simulink model "Trajactory_uav"  (R2022a)
settings: Solver=ode4  StartTime=0.0  StopTime=25  FixedStep=0.01  RelTol=1e-3
settings Model: Creator=liuwhale  LastModifiedBy=liuwhale
settings DebuggingCC: UnconnectedInputMsg=warning  UnconnectedOutputMsg=warning  UnconnectedLineMsg=warning
settings RTWCC: DLArmComputeVersion=19.05

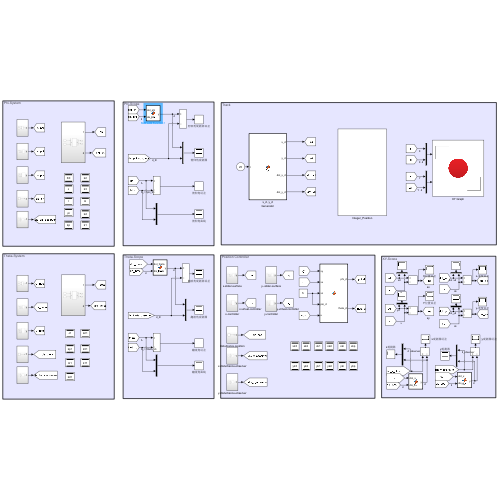
[thumbnail: Simulink's stored preview of the top-level diagram]
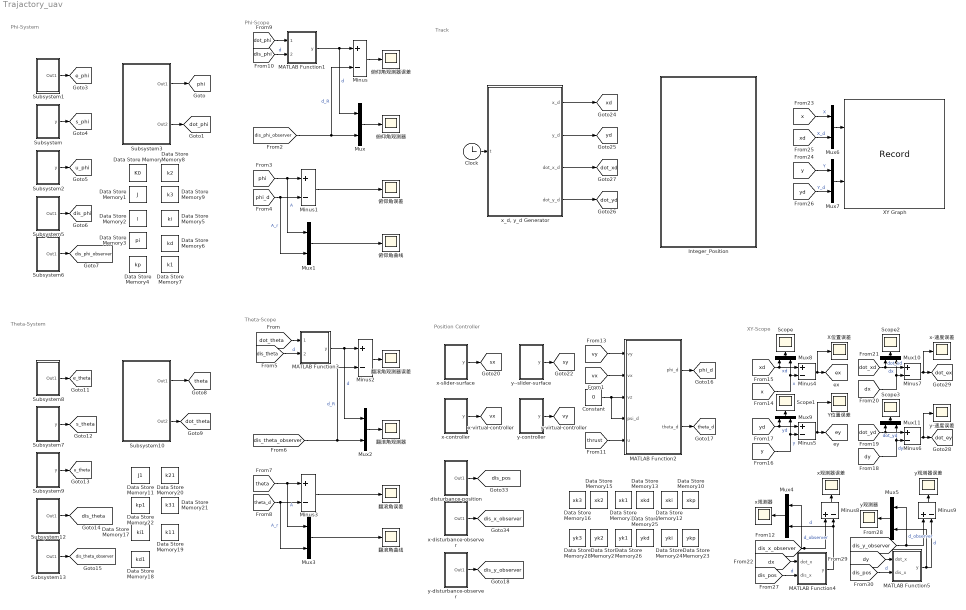
== system Trajactory_uav ==
  note: XY-Scope
  note: Track
  note: Position Controller
  note: Phi-Scope
  note: Phi-System
  note: Theta-System
  note: Theta-Scope
  Clock : Clock
  Constant : Constant  Value=0
  Data Store Memory : DataStoreMemory  DataStoreName=K0  ReadBeforeWriteMsg=warning  WriteAfterWriteMsg=warning  WriteAfterReadMsg=warning  InitialValue=0.01  ShowAdditionalParam=off  OutDataTypeStr=double
  Data Store Memory1 : DataStoreMemory  DataStoreName=J  ReadBeforeWriteMsg=warning  WriteAfterWriteMsg=warning  WriteAfterReadMsg=warning  InitialValue=0.005309688  ShowAdditionalParam=off  OutDataTypeStr=double
  Data Store Memory10 : DataStoreMemory  DataStoreName=xkp  ReadBeforeWriteMsg=warning  WriteAfterWriteMsg=warning  WriteAfterReadMsg=warning  InitialValue=1  ShowAdditionalParam=off  OutDataTypeStr=double
  Data Store Memory11 : DataStoreMemory  DataStoreName=J1  ReadBeforeWriteMsg=warning  WriteAfterWriteMsg=warning  WriteAfterReadMsg=warning  InitialValue=0.00577  ShowAdditionalParam=off  OutDataTypeStr=double
  Data Store Memory12 : DataStoreMemory  DataStoreName=xki  ReadBeforeWriteMsg=warning  WriteAfterWriteMsg=warning  WriteAfterReadMsg=warning  ShowAdditionalParam=off  OutDataTypeStr=double
  Data Store Memory13 : DataStoreMemory  DataStoreName=xkd  ReadBeforeWriteMsg=warning  WriteAfterWriteMsg=warning  WriteAfterReadMsg=warning  InitialValue=1  ShowAdditionalParam=off  OutDataTypeStr=double
  Data Store Memory14 : DataStoreMemory  DataStoreName=xk1  ReadBeforeWriteMsg=warning  WriteAfterWriteMsg=warning  WriteAfterReadMsg=warning  InitialValue=1  ShowAdditionalParam=off  OutDataTypeStr=double
  Data Store Memory15 : DataStoreMemory  DataStoreName=xk2  ReadBeforeWriteMsg=warning  WriteAfterWriteMsg=warning  WriteAfterReadMsg=warning  InitialValue=100  ShowAdditionalParam=off  OutDataTypeStr=double
  Data Store Memory16 : DataStoreMemory  DataStoreName=xk3  ReadBeforeWriteMsg=warning  WriteAfterWriteMsg=warning  WriteAfterReadMsg=warning  ShowAdditionalParam=off  OutDataTypeStr=double
  Data Store Memory17 : DataStoreMemory  DataStoreName=ki1  ReadBeforeWriteMsg=warning  WriteAfterWriteMsg=warning  WriteAfterReadMsg=warning  InitialValue=0.01  ShowAdditionalParam=off  OutDataTypeStr=double
  Data Store Memory18 : DataStoreMemory  DataStoreName=kd1  ReadBeforeWriteMsg=warning  WriteAfterWriteMsg=warning  WriteAfterReadMsg=warning  InitialValue=1  ShowAdditionalParam=off  OutDataTypeStr=double
  Data Store Memory19 : DataStoreMemory  DataStoreName=k11  ReadBeforeWriteMsg=warning  WriteAfterWriteMsg=warning  WriteAfterReadMsg=warning  InitialValue=1  ShowAdditionalParam=off  OutDataTypeStr=double
  Data Store Memory2 : DataStoreMemory  DataStoreName=l  ReadBeforeWriteMsg=warning  WriteAfterWriteMsg=warning  WriteAfterReadMsg=warning  InitialValue=0.33/sqrt(2)  ShowAdditionalParam=off  OutDataTypeStr=double
  Data Store Memory20 : DataStoreMemory  DataStoreName=k21  ReadBeforeWriteMsg=warning  WriteAfterWriteMsg=warning  WriteAfterReadMsg=warning  InitialValue=5  ShowAdditionalParam=off  OutDataTypeStr=double
  Data Store Memory21 : DataStoreMemory  DataStoreName=k31  ReadBeforeWriteMsg=warning  WriteAfterWriteMsg=warning  WriteAfterReadMsg=warning  InitialValue=0.001  ShowAdditionalParam=off  OutDataTypeStr=double
  Data Store Memory22 : DataStoreMemory  DataStoreName=kp1  ReadBeforeWriteMsg=warning  WriteAfterWriteMsg=warning  WriteAfterReadMsg=warning  InitialValue=30  ShowAdditionalParam=off  OutDataTypeStr=double
  Data Store Memory23 : DataStoreMemory  DataStoreName=ykp  ReadBeforeWriteMsg=warning  WriteAfterWriteMsg=warning  WriteAfterReadMsg=warning  InitialValue=1  ShowAdditionalParam=off  OutDataTypeStr=double
  Data Store Memory24 : DataStoreMemory  DataStoreName=yki  ReadBeforeWriteMsg=warning  WriteAfterWriteMsg=warning  WriteAfterReadMsg=warning  ShowAdditionalParam=off  OutDataTypeStr=double
  Data Store Memory25 : DataStoreMemory  DataStoreName=ykd  ReadBeforeWriteMsg=warning  WriteAfterWriteMsg=warning  WriteAfterReadMsg=warning  InitialValue=1  ShowAdditionalParam=off  OutDataTypeStr=double
  Data Store Memory26 : DataStoreMemory  DataStoreName=yk1  ReadBeforeWriteMsg=warning  WriteAfterWriteMsg=warning  WriteAfterReadMsg=warning  InitialValue=1  ShowAdditionalParam=off  OutDataTypeStr=double
  Data Store Memory27 : DataStoreMemory  DataStoreName=yk2  ReadBeforeWriteMsg=warning  WriteAfterWriteMsg=warning  WriteAfterReadMsg=warning  InitialValue=100  ShowAdditionalParam=off  OutDataTypeStr=double
  Data Store Memory28 : DataStoreMemory  DataStoreName=yk3  ReadBeforeWriteMsg=warning  WriteAfterWriteMsg=warning  WriteAfterReadMsg=warning  ShowAdditionalParam=off  OutDataTypeStr=double
  Data Store Memory3 : DataStoreMemory  DataStoreName=pi  ReadBeforeWriteMsg=warning  WriteAfterWriteMsg=warning  WriteAfterReadMsg=warning  InitialValue=3.1415926  ShowAdditionalParam=off  OutDataTypeStr=double
  Data Store Memory4 : DataStoreMemory  DataStoreName=kp  ReadBeforeWriteMsg=warning  WriteAfterWriteMsg=warning  WriteAfterReadMsg=warning  InitialValue=30  ShowAdditionalParam=off  OutDataTypeStr=double
  Data Store Memory5 : DataStoreMemory  DataStoreName=ki  ReadBeforeWriteMsg=warning  WriteAfterWriteMsg=warning  WriteAfterReadMsg=warning  InitialValue=0.01  ShowAdditionalParam=off  OutDataTypeStr=double
  Data Store Memory6 : DataStoreMemory  DataStoreName=kd  ReadBeforeWriteMsg=warning  WriteAfterWriteMsg=warning  WriteAfterReadMsg=warning  InitialValue=1  ShowAdditionalParam=off  OutDataTypeStr=double
  Data Store Memory7 : DataStoreMemory  DataStoreName=k1  ReadBeforeWriteMsg=warning  WriteAfterWriteMsg=warning  WriteAfterReadMsg=warning  InitialValue=1  ShowAdditionalParam=off  OutDataTypeStr=double
  Data Store Memory8 : DataStoreMemory  DataStoreName=k2  ReadBeforeWriteMsg=warning  WriteAfterWriteMsg=warning  WriteAfterReadMsg=warning  InitialValue=5  ShowAdditionalParam=off  OutDataTypeStr=double
  Data Store Memory9 : DataStoreMemory  DataStoreName=k3  ReadBeforeWriteMsg=warning  WriteAfterWriteMsg=warning  WriteAfterReadMsg=warning  InitialValue=0.001  ShowAdditionalParam=off  OutDataTypeStr=double
  Integer_Position : Subsystem
  MATLAB Function1 : MATLAB Function  TreatAsAtomicUnit=on
  MATLAB Function2 : MATLAB Function  TreatAsAtomicUnit=on
  MATLAB Function3 : MATLAB Function  TreatAsAtomicUnit=on
  MATLAB Function4 : MATLAB Function  TreatAsAtomicUnit=on
  MATLAB Function5 : MATLAB Function  TreatAsAtomicUnit=on
  Minus{,1..9} (10 alike) : Sum  Inputs=+-
  Mux{,1..11} (12 alike) : Mux  Inputs=2
  Scope{,1..3} (4 alike) : Scope
  Subsystem : Subsystem
  Subsystem1 : Subsystem
  Subsystem10 : Subsystem
  Subsystem12 : Subsystem
  Subsystem13 : Subsystem
  Subsystem2 : Subsystem
  Subsystem3 : Subsystem
  Subsystem5 : Subsystem
  Subsystem6 : Subsystem
  Subsystem7 : Subsystem
  Subsystem8 : Subsystem
  Subsystem9 : Subsystem
  XY Graph : Record  RecordToWorkspace=on  FileSettingsInternal="{\"entries\":[{\"content\":{\"excelSettings\":{\"content\":{},\"type\":\"Streamout.ExcelSettings\"}},\"type\":\"Streamout.FileSettingStorage\",\"uuid\":\"cb515a56-81c6-47bd-8ef5-eec051ca2d3d\"}],\"packageUris\":[\"http://schema.mathworks.com/mf0/streamout_blocks/R2020a\"],\"version\":\"1.0\"}"  Layout=[1 1]  SignalsInternal="{\"entries\":[{\"content\":{\"signals\":[{\"content\":{\"blockPath\":[\"Trajactory_uav/XY Graph\"],\"channel\":[],\"dimensions\":[2],\"domain\":\"Trajactory_uav/XY Graph\",\"hasChildren\":true,\"lineColor\":\"#0072bd\",\"plots\":[],\"port\":1,\"sid\":[\"\"],\"signalID\":412,\"signalName\":\"Mux6\"},\"type\":\"RecordBlkView.Signal\",\"uuid\":\"3dcd1e12-03f3-405f-916b-5c80faeb8bef\"},{\"content\":{\"blockPath\":[\"Trajactory_uav/XY Graph\"],\"channel\":[1],\"dimensions\":[2],\"domain\":\"Trajactory_uav/XY Graph\",\"lineColor\":\"#d95319\",\"parentID\":412,\"plots\":[1],\"port\":1,\"sid\":[\"\"],\"signalID\":413,\"signalName\":\"Mux6\"},\"type\":\"RecordBlkView.Signal\",\"uuid\":\"11d0947b-d576-4e4d-964d-e577cf2fd32e\"},{\"content\":{\"blockPath\":[\"Trajactory_uav/XY Graph\"],\"channel\":[],\"dimensions\":[2],\"domain\":\"Trajactory_uav/XY Graph\",\"hasChildren\":true,\"lineColor\":\"#edb120\",\"plots\":[],\"port\":2,\"sid\":[\"\"],\"signalID\":417,\"signalName\":\"Mux7\"},\"type\":\"RecordBlkView.Signal\",\"uuid\":\"3379d438-6583-47b9-80cc-092c1c32a13f\"},{\"content\":{\"blockPath\":[\"Trajactory_uav/XY Graph\"],\"channel\":[1],\"dimensions\":[2],\"domain\":\"Trajactory_uav/XY Graph\",\"lineColor\":\"#0072bd\",\"parentID\":417,\"plots\":[1],\"port\":2,\"sid\":[\"\"],\"signalID\":418,\"signalName\":\"Mux7\"},\"type\":\"RecordBlkView.Signal\",\"uuid\":\"342c55b0-3c25-4b78-9321-4ec9a5f92615\"},{\"content\":{\"blockPath\":[\"Trajactory_uav/XY Graph\"],\"channel\":[2],\"dimensions\":[2],\"domain\":\"Trajactory_uav/XY Graph\",\"lineColor\":\"#ff6929\",\"parentID\":412,\"plots\":[1],\"port\":1,\"sid\":[\"\"],\"signalID\":431,\"signalName\":\"Mux6\"},\"type\":\"RecordBlkView.Signal\",\"uuid\":\"21f03ca2-9128-487a-99db-9b74c0302f26\"},{\"content\":{\"blockPath\":[\"Trajactory_uav/XY Graph\"],\"channel\":[2],\"dimensions\":[2],\"domain\":\"Trajactory_uav/XY Graph\",\"lineColor\":\"#d95319\",\"parentID\":417,\"plots\":[1],\"port\":2,\"sid\":[\"\"],\"signalID\":432,\"signalName\":\"Mux7\"},\"type\":\"RecordBlkView.Signal\",\"uuid\":\"e9a965a2-3574-4d7b-b30c-2ed9b65f5195\"}]},\"type\":\"RecordBlkView.InputSignals\",\"uuid\":\"7f01d153-5e7e-44f9-865f-c21572bec30b\"}],\"packageUris\":[\"http://schema.mathworks.com/mf0/streamout_blocks/R2020a\"],\"version\":\"1.0\"}"  VisualizationBindings="{\"xyplotplugin\":{\"info\":[{\"series\":[{\"bindingParametersList\":[{\"parameter\":\"X-Axis\",\"signalID\":413,\"signalName\":\"Mux6(1)\"},{\"parameter\":\"Y-Axis\",\"signalID\":418,\"signalName\":\"Mux7(1)\"}],\"seriesID\":8627},{\"bindingParametersList\":[{\"parameter\":\"X-Axis\",\"signalID\":431,\"signalName\":\"Mux6(2)\"},{\"parameter\":\"Y-Axis\",\"signalID\":432,\"signalName\":\"Mux7(2)\"}],\"seriesID\":43199}],\"subplotID\":1}]}}"  CompatibilityTag=XY
  X位置误差 : Scope
  Y位置误差 : Scope
  disturbance-position : Subsystem
  x-controller : Subsystem
  x-disturbance-observer : Subsystem
  x-slider-surface : Subsystem
  x-速度误差 : Scope
  "x_d, y_d Generator" : MATLAB Function  TreatAsAtomicUnit=on
  x观测器 : Scope
  x观测器误差 : Scope
  y--slider-surface : Subsystem
  y-controller : Subsystem
  y-disturbance-observer : Subsystem
  y-速度误差 : Scope
  y观测器 : Scope
  y观测器误差 : Scope
  俯仰角曲线 : Scope
  俯仰角观测器 : Scope
  俯仰角观测器误差 : Scope
  俯仰角误差 : Scope
  翻滚角曲线 : Scope
  翻滚角观测器 : Scope
  翻滚角观测器误差 : Scope
  翻滚角误差 : Scope
  tag scope: dis_phi=global, dis_phi_observer=global, dis_pos=global, dis_theta=global, dis_theta_observer=global, dis_x_observer=global, dis_y_observer=global, dot_ex=global, dot_ey=global, dot_phi=global, dot_theta=global, dot_xd=global, dot_yd=global, e_phi=global, e_theta=global, ex=global, ey=global, phi=global, phi_d=global, s_phi=global, s_theta=global, sx=global, sy=global, theta=global, theta_d=global, u_phi=global, u_theta=global, vx=global, vy=global, xd=global, yd=global
  wires:
  Subsystem/1(y) -> [s_phi]
  Subsystem1/1(Out1) -> [e_phi]
  Subsystem2/1(y) -> [u_phi]
  Subsystem3/2(Out2) -> [dot_phi]
  Subsystem5/1(Out1) -> [dis_phi]
  Subsystem6/1(Out1) -> [dis_phi_observer]
  MATLAB Function1/1(y) -> Mux/1, Minus/1  "d"
  [dis_phi_observer] -> Minus/2, Mux/2  "d_R"
  Minus/1 -> 俯仰角观测器误差/1
  Mux/1 -> 俯仰角观测器/1
  Minus1/1 -> 俯仰角误差/1
  Mux1/1 -> 俯仰角曲线/1
  [phi_d] -> Mux1/2, Minus1/2  "A_r"
  [phi] -> Mux1/1, Minus1/1  "A"
  Subsystem8/1(Out1) -> [e_theta]
  Subsystem12/1(Out1) -> [dis_theta]
  Subsystem13/1(Out1) -> [dis_theta_observer]
  Subsystem7/1(y) -> [s_theta]
  Subsystem10/2(Out2) -> [dot_theta]
  Subsystem9/1(y) -> [u_theta]
  Minus2/1 -> 翻滚角观测器误差/1
  [theta] -> Mux3/1, Minus3/1  "A"
  [dis_theta_observer] -> Minus2/2, Mux2/2  "d_R"
  MATLAB Function3/1(y) -> Mux2/1, Minus2/1  "d"
  [theta_d] -> Mux3/2, Minus3/2  "A_r"
  Minus3/1 -> 翻滚角误差/1
  Mux3/1 -> 翻滚角曲线/1
  Mux2/1 -> 翻滚角观测器/1
  [dot_theta] -> MATLAB Function3/1(dot_theta)
  [dis_phi] -> MATLAB Function1/2(dis_phi)  "d"
  [dot_phi] -> MATLAB Function1/1(dot_phi)
  "x_d, y_d Generator"/2(y_d) -> [yd]
  "x_d, y_d Generator"/4(dot_y_d) -> [dot_yd]
  "x_d, y_d Generator"/3(dot_x_d) -> [dot_xd]
  Subsystem3/1(Out1) -> [phi]
  Subsystem10/1(Out1) -> [theta]
  Minus5/1 -> Y位置误差/1, [ey]
  [yd] -> Mux9/1, Minus5/1  "yd"
  [dx] -> Mux10/2, Minus7/2  "dx"
  [dy] -> Mux11/2, Minus6/2  "dy"
  Minus7/1 -> x-速度误差/1, [dot_ex]
  [x] -> Mux8/2, Minus4/2  "x"
  [dot_xd] -> Minus7/1, Mux10/1  "dot_xd"
  Minus6/1 -> y-速度误差/1, [dot_ey]
  [xd] -> Minus4/1, Mux8/1  "xd"
  Minus4/1 -> X位置误差/1, [ex]
  [dot_yd] -> Mux11/1, Minus6/1  "dot_yd"
  MATLAB Function2/2(theta_d) -> [theta_d]
  MATLAB Function2/1(phi_d) -> [phi_d]
  [thrust] -> MATLAB Function2/5(u)
  Constant/1 -> MATLAB Function2/3(vz), MATLAB Function2/4(psi_d)
  y-controller/1(y) -> [vy]
  x-controller/1(y) -> [vx]
  y--slider-surface/1(y) -> [sy]
  x-slider-surface/1(y) -> [sx]
  Clock/1 -> "x_d, y_d Generator"/1(t)
  "x_d, y_d Generator"/1(x_d) -> [xd]
  [vy] -> MATLAB Function2/1(vy)
  [vx] -> MATLAB Function2/2(vx)
  [dis_theta] -> MATLAB Function3/2(dis_theta)  "d"
  x-disturbance-observer/1(Out1) -> [dis_x_observer]
  disturbance-position/1(Out1) -> [dis_pos]
  [dx] -> MATLAB Function4/1(dot_x)
  [dis_x_observer] -> Minus8/1, Mux4/1  "d_observer"
  Mux4/1 -> x观测器/1
  MATLAB Function4/1(y) -> Mux4/2, Minus8/2  "d"
  Minus8/1 -> x观测器误差/1
  [dis_pos] -> MATLAB Function4/2(dis_x)  "d"
  y-disturbance-observer/1(Out1) -> [dis_y_observer]
  [dis_pos] -> MATLAB Function5/2(dis_x)  "d"
  [dy] -> MATLAB Function5/1(dot_x)
  MATLAB Function5/1(y) -> Minus9/2, Mux5/2  "d"
  Mux5/1 -> y观测器/1
  [dis_y_observer] -> Minus9/1, Mux5/1  "d_observer"
  Minus9/1 -> y观测器误差/1
  [yd] -> Mux7/2  "Y_d"
  Mux7/1 -> XY Graph/2
  [y] -> Mux7/1  "Y"
  Mux6/1 -> XY Graph/1
  [xd] -> Mux6/2  "X_d"
  [x] -> Mux6/1  "X"
  Mux8/1 -> Scope/1
  Mux9/1 -> Scope1/1
  [y] -> Mux9/2, Minus5/2  "y"
  Mux10/1 -> Scope2/1
  Mux11/1 -> Scope3/1

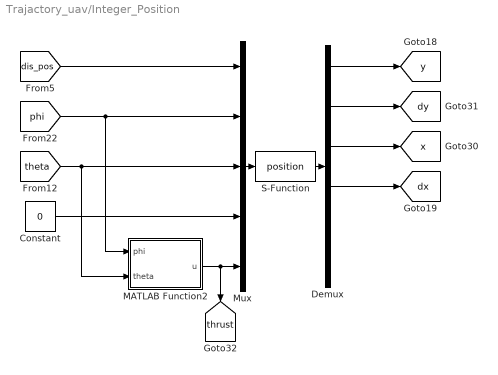
== system Trajactory_uav/Integer_Position ==
  Constant : Constant  Value=0
  Demux : Demux  Outputs=6
  MATLAB Function2 : MATLAB Function  TreatAsAtomicUnit=on
  Mux : Mux  Inputs=5
  S-Function : S-Function  FunctionName=position  SFunctionDeploymentMode=off  EnableBusSupport=off
  tag scope: dx=global, dy=global, thrust=global, x=global, y=global
  wires:
  [theta] -> Mux/3, MATLAB Function2/2(theta)
  [phi] -> Mux/2, MATLAB Function2/1(phi)
  MATLAB Function2/1(u) -> [thrust], Mux/5
  Mux/1 -> S-Function/1
  S-Function/1 -> Demux/1
  Constant/1 -> Mux/4
  Demux/3 -> [x]
  Demux/1 -> [y]
  Demux/2 -> [dy]
  Demux/4 -> [dx]
  [dis_pos] -> Mux/1

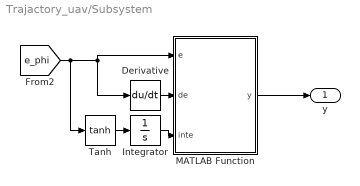
== system Trajactory_uav/Subsystem ==
  Derivative : Derivative
  Integrator : Integrator
  MATLAB Function : MATLAB Function  TreatAsAtomicUnit=on
  Tanh : Trigonometry  Operator=tanh
  y : Outport
  wires:
  [e_phi] -> Tanh/1, Derivative/1, MATLAB Function/1(e)
  Derivative/1 -> MATLAB Function/2(de)
  Integrator/1 -> MATLAB Function/3(inte)
  MATLAB Function/1(y) -> y/1
  Tanh/1 -> Integrator/1

== system Trajactory_uav/Subsystem1 ==
  Minus : Sum  Inputs=-+
  Out1 : Outport
  wires:
  [phi] -> Minus/1
  [phi_d] -> Minus/2
  Minus/1 -> Out1/1

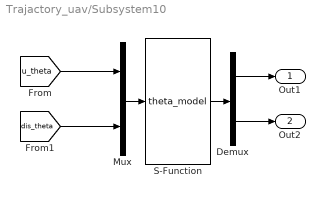
== system Trajactory_uav/Subsystem10 ==
  Demux : Demux  Outputs=2
  Mux : Mux  Inputs=2
  S-Function : S-Function  FunctionName=theta_model  SFunctionDeploymentMode=off  EnableBusSupport=off
  Out1 : Outport
  Out2 : Outport  Port=2
  wires:
  Mux/1 -> S-Function/1
  [u_theta] -> Mux/1
  S-Function/1 -> Demux/1
  Demux/1 -> Out1/1
  Demux/2 -> Out2/1
  [dis_theta] -> Mux/2

== system Trajactory_uav/Subsystem12 ==
  Sine Wave : Sin  Frequency=100  SampleTime=0
  Out1 : Outport
  wires:
  Sine Wave/1 -> Out1/1

== system Trajactory_uav/Subsystem13 ==
  Mux : Mux  Inputs=2
  S-Function : S-Function  FunctionName=DO_theta  SFunctionDeploymentMode=off  EnableBusSupport=off
  Out1 : Outport
  wires:
  S-Function/1 -> Out1/1
  [u_theta] -> Mux/1
  [dot_theta] -> Mux/2
  Mux/1 -> S-Function/1

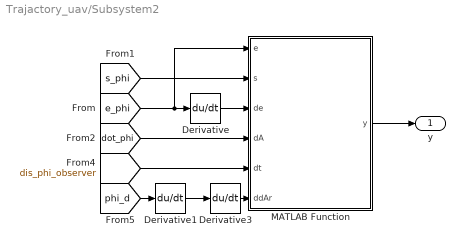
== system Trajactory_uav/Subsystem2 ==
  Derivative : Derivative
  Derivative1 : Derivative
  Derivative3 : Derivative
  MATLAB Function : MATLAB Function  TreatAsAtomicUnit=on
  y : Outport
  wires:
  [phi_d] -> Derivative1/1
  [s_phi] -> MATLAB Function/2(s)
  Derivative3/1 -> MATLAB Function/6(ddAr)
  [e_phi] -> MATLAB Function/1(e), Derivative/1
  MATLAB Function/1(y) -> y/1
  [dot_phi] -> MATLAB Function/4(dA)
  Derivative/1 -> MATLAB Function/3(de)
  Derivative1/1 -> Derivative3/1
  [dis_phi_observer] -> MATLAB Function/5(dt)

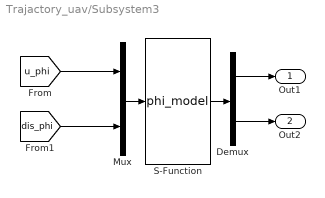
== system Trajactory_uav/Subsystem3 ==
  Demux : Demux  Outputs=2
  Mux : Mux  Inputs=2
  S-Function : S-Function  FunctionName=phi_model  SFunctionDeploymentMode=off  EnableBusSupport=off
  Out1 : Outport
  Out2 : Outport  Port=2
  wires:
  Mux/1 -> S-Function/1
  [u_phi] -> Mux/1
  S-Function/1 -> Demux/1
  Demux/1 -> Out1/1
  Demux/2 -> Out2/1
  [dis_phi] -> Mux/2

== system Trajactory_uav/Subsystem5 ==
  Sine Wave : Sin  Frequency=100  SampleTime=0
  Out1 : Outport
  wires:
  Sine Wave/1 -> Out1/1

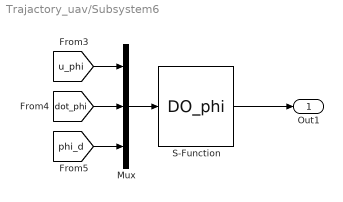
== system Trajactory_uav/Subsystem6 ==
  Mux : Mux  Inputs=3
  S-Function : S-Function  FunctionName=DO_phi  SFunctionDeploymentMode=off  EnableBusSupport=off
  Out1 : Outport
  wires:
  S-Function/1 -> Out1/1
  [u_phi] -> Mux/1
  [phi_d] -> Mux/3
  [dot_phi] -> Mux/2
  Mux/1 -> S-Function/1

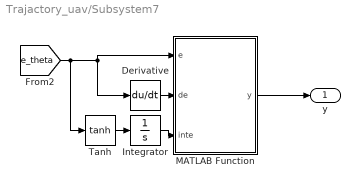
== system Trajactory_uav/Subsystem7 ==
  Derivative : Derivative
  Integrator : Integrator
  MATLAB Function : MATLAB Function  TreatAsAtomicUnit=on
  Tanh : Trigonometry  Operator=tanh
  y : Outport
  wires:
  [e_theta] -> Tanh/1, Derivative/1, MATLAB Function/1(e)
  Derivative/1 -> MATLAB Function/2(de)
  Integrator/1 -> MATLAB Function/3(inte)
  MATLAB Function/1(y) -> y/1
  Tanh/1 -> Integrator/1

== system Trajactory_uav/Subsystem8 ==
  Minus : Sum  Inputs=-+
  Out1 : Outport
  wires:
  [theta] -> Minus/1
  [theta_d] -> Minus/2
  Minus/1 -> Out1/1

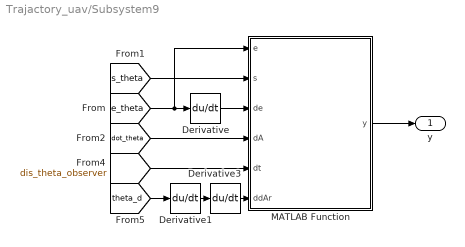
== system Trajactory_uav/Subsystem9 ==
  Derivative : Derivative
  Derivative1 : Derivative
  Derivative3 : Derivative
  MATLAB Function : MATLAB Function  TreatAsAtomicUnit=on
  y : Outport
  wires:
  [theta_d] -> Derivative1/1
  [s_theta] -> MATLAB Function/2(s)
  Derivative3/1 -> MATLAB Function/6(ddAr)
  [e_theta] -> MATLAB Function/1(e), Derivative/1
  MATLAB Function/1(y) -> y/1
  Derivative/1 -> MATLAB Function/3(de)
  Derivative1/1 -> Derivative3/1
  [dis_theta_observer] -> MATLAB Function/5(dt)
  [dot_theta] -> MATLAB Function/4(dA)

== system Trajactory_uav/disturbance-position ==
  Sine Wave : Sin  SampleTime=0
  Out1 : Outport
  wires:
  Sine Wave/1 -> Out1/1

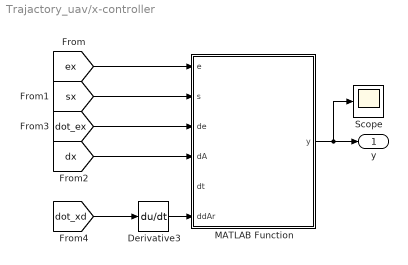
== system Trajactory_uav/x-controller ==
  Derivative3 : Derivative
  MATLAB Function : MATLAB Function  TreatAsAtomicUnit=on
  Scope : Scope
  y : Outport
  wires:
  [dx] -> MATLAB Function/4(dA)
  [sx] -> MATLAB Function/2(s)
  Derivative3/1 -> MATLAB Function/6(ddAr)
  [ex] -> MATLAB Function/1(e)
  MATLAB Function/1(y) -> Scope/1, y/1
  [dot_ex] -> MATLAB Function/3(de)
  ? -> MATLAB Function/5(dt)
  [dot_xd] -> Derivative3/1

== system Trajactory_uav/x-disturbance-observer ==
  Mux : Mux  Inputs=2
  S-Function : S-Function  FunctionName=DO_x  SFunctionDeploymentMode=off  EnableBusSupport=off
  Out1 : Outport
  wires:
  S-Function/1 -> Out1/1
  [vx] -> Mux/1
  [dx] -> Mux/2
  Mux/1 -> S-Function/1

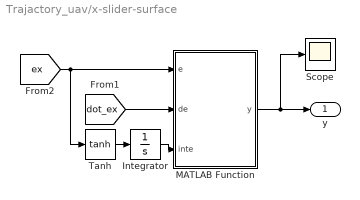
== system Trajactory_uav/x-slider-surface ==
  Integrator : Integrator
  MATLAB Function : MATLAB Function  TreatAsAtomicUnit=on
  Scope : Scope
  Tanh : Trigonometry  Operator=tanh
  y : Outport
  wires:
  [ex] -> Tanh/1, MATLAB Function/1(e)
  [dot_ex] -> MATLAB Function/2(de)
  Integrator/1 -> MATLAB Function/3(inte)
  MATLAB Function/1(y) -> Scope/1, y/1
  Tanh/1 -> Integrator/1

== system Trajactory_uav/y--slider-surface ==
  Integrator : Integrator
  MATLAB Function : MATLAB Function  TreatAsAtomicUnit=on
  Tanh : Trigonometry  Operator=tanh
  y : Outport
  wires:
  [ey] -> Tanh/1, MATLAB Function/1(e)
  [dot_ey] -> MATLAB Function/2(de)
  Integrator/1 -> MATLAB Function/3(inte)
  MATLAB Function/1(y) -> y/1
  Tanh/1 -> Integrator/1

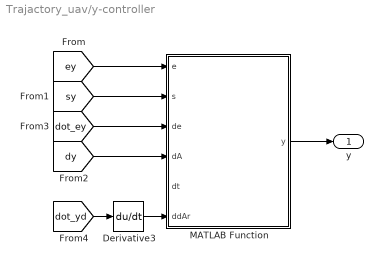
== system Trajactory_uav/y-controller ==
  Derivative3 : Derivative
  MATLAB Function : MATLAB Function  TreatAsAtomicUnit=on
  y : Outport
  wires:
  [dy] -> MATLAB Function/4(dA)
  [sy] -> MATLAB Function/2(s)
  Derivative3/1 -> MATLAB Function/6(ddAr)
  [ey] -> MATLAB Function/1(e)
  MATLAB Function/1(y) -> y/1
  [dot_ey] -> MATLAB Function/3(de)
  ? -> MATLAB Function/5(dt)
  [dot_yd] -> Derivative3/1

== system Trajactory_uav/y-disturbance-observer ==
  Mux : Mux  Inputs=2
  S-Function : S-Function  FunctionName=DO_x  SFunctionDeploymentMode=off  EnableBusSupport=off
  Out1 : Outport
  wires:
  S-Function/1 -> Out1/1
  [vy] -> Mux/1
  [dy] -> Mux/2
  Mux/1 -> S-Function/1

== matlab function Trajactory_uav/x-controller/MATLAB Function ==
  settings: updateMethod=DISCRETE
  data: e input; s input; y output; de input; dA input; dt input; ddAr input; K0 data_store_memory; J data_store_memory; l data_store_memory; pi data_store_memory; xkp data_store_memory; xki data_store_memory; xk1 data_store_memory; xk2 data_store_memory; xk3 data_store_memory; xkd data_store_memory
function y = fcn(e,s,de,dA,dt,ddAr)
global xkp xki xkd xk1 xk2 xk3;

y =-dt+ddAr+1/xkd*(xkp*de+xki*xk1*tanh(e)+xk2*s+xk3*sign(s));

== matlab function Trajactory_uav/Integer_Position/MATLAB Function2 ==
  data: phi input; u output; theta input
function u = fcn(phi,theta)
m = 1;
g = 9.8;
u =m*g/(cos(theta)*cos(phi)) ;

== matlab function Trajactory_uav/x_d, y_d Generator ==
  data: x_d output; y_d output; t input; dot_x_d output; dot_y_d output
function [x_d, y_d, dot_x_d, dot_y_d] = fcn(t)
%--------------------------------------------------------------------------
% Set Parameters:
pi = 3.14159265358;
% A1_X = 2;        A1_Y = 2;
% A2_X = 1;        A2_Y = 1;
% tr_X = 8;        tr_Y = 8;
% w2_X = 2*pi;     w2_Y = 2.5*pi;
r=2;
T=50;
omega=2*pi/T;
t_f=T/4;
%--------------------------------------------------------------------------
% Define temp of outputs
o_X = 0;         o_Y = 0;
dot_o_X  = 0;    dot_o_Y  = 0;
%--------------------------------------------------------------------------
% Construct outputs:
n = 1;
switch n
    case 1
%         if t<tr_X
%             o_X = -(A1_X/2)*cos((pi/tr_X)*t) + A1_X/2;
%             dot_o_X  = (pi/tr_X)*(A1_X/2)*sin((pi/tr_X)*t);
%             
%         elseif t>=tr_X
%             o_X = (A2_X/2)*cos((2*pi/w2_X)*(t-tr_X)) + A1_X - A2_X/2;
%             dot_o_X  = -(2*pi/w2_X)*(A2_X/2)*sin((2*pi/w2_X)*(t-tr_X));
%            
%         end
% 
%         if t<tr_Y
%             o_Y = -(A1_Y/2)*cos((pi/tr_Y)*t) + A1_Y/2;
%             dot_o_Y  = (pi/tr_Y)*(A1_Y/2)*sin((pi/tr_Y)*t);     
%             
%         elseif t>=tr_Y
%             o_Y = (A2_Y/2)*cos((2*pi/w2_Y)*(t-tr_Y)) + A1_Y - A2_Y/2;
%             dot_o_Y  = -(2*pi/w2_Y)*(A2_Y/2)*sin((2*pi/w2_Y)*(t-tr_Y));
%             
%         end
%         o_X = t;
%         dot_o_X = 1;
%         o_Y = t;
%         dot_o_Y = 1;
        o_Y = r*sin(2*omega*t);
        dot_o_Y = 2*omega*r*cos(2*omega*t);
        o_X=2*r*sin(omega*t)*sin(omega*t);
        dot_o_X=2*omega*r*sin(2*omega*t);
        
    case 2
        o_X = 0;
        dot_o_X  = 0;
       
end
%--------------------------------------------------------------------------
% Output:
x_d = o_X;
dot_x_d = dot_o_X;


y_d = o_Y;
dot_y_d = dot_o_Y;

%--------------------------------------------------------------------------

== matlab function Trajactory_uav/MATLAB Function2 ==
  data: vy input; vx input; phi_d output; vz input; psi_d input; theta_d output; u input
function [phi_d,theta_d] = fcn(vy,vx,vz,psi_d,u)
g = 9.8;
c = (vy*sin(psi_d)-vx*cos(psi_d))/u;
if abs(c) <= 1
    a = asin(c);
else
    a = asin(abs(c)/c*1);
end
b = atan((vy*cos(psi_d)+vx*sin(psi_d))/(g-vz));

phi_d = a;
theta_d = b;

== matlab function Trajactory_uav/y--slider-surface/MATLAB Function ==
  settings: updateMethod=DISCRETE
  data: e input; y output; de input; inte input; ykp data_store_memory; yki data_store_memory; yk1 data_store_memory; yk2 data_store_memory; yk3 data_store_memory; ykd data_store_memory
function y = fcn(e,de,inte)
global ykp;
global yki;
global ykd;
global yk1;

y = ykp*e+yki*yk1*inte+ykd*de;

== matlab function Trajactory_uav/y-controller/MATLAB Function ==
  settings: updateMethod=DISCRETE
  data: e input; s input; y output; de input; dA input; dt input; ddAr input; K0 data_store_memory; J data_store_memory; l data_store_memory; pi data_store_memory; ykp data_store_memory; yki data_store_memory; yk1 data_store_memory; yk2 data_store_memory; yk3 data_store_memory; ykd data_store_memory
function y = fcn(e,s,de,dA,dt,ddAr)
global ykp yki ykd yk1 yk2 yk3;

y =-dt+ddAr+1/ykd*(ykp*de+yki*yk1*tanh(e)+yk2*s+yk3*sign(s));

== matlab function Trajactory_uav/MATLAB Function3 ==
  settings: updateMethod=DISCRETE  sampleTime=0.01
  data: dot_theta input; y output; l data_store_memory; K0 data_store_memory; dis_theta input
function y = fcn(dot_theta,dis_theta)
global l K0;
y = -l*K0*dot_theta+dis_theta;

== matlab function Trajactory_uav/MATLAB Function1 ==
  settings: updateMethod=DISCRETE  sampleTime=0.01
  data: dot_phi input; y output; l data_store_memory; K0 data_store_memory; dis_phi input
function y = fcn(dot_phi,dis_phi)
global l K0;
y = -l*K0*dot_phi+dis_phi;

== matlab function Trajactory_uav/MATLAB Function4 ==
  settings: updateMethod=DISCRETE  sampleTime=0.01
  data: dot_x input; y output; l data_store_memory; K0 data_store_memory; dis_x input
function y = fcn(dot_x,dis_x)
global K0;
y = -K0*dot_x+dis_x;

== matlab function Trajactory_uav/MATLAB Function5 ==
  settings: updateMethod=DISCRETE  sampleTime=0.01
  data: dot_x input; y output; l data_store_memory; K0 data_store_memory; dis_x input
function y = fcn(dot_x,dis_x)
global K0;
y = -K0*dot_x+dis_x;

== matlab function Trajactory_uav/Subsystem2/MATLAB Function ==
  settings: updateMethod=DISCRETE
  data: e input; s input; y output; de input; dA input; dt input; ddAr input; K0 data_store_memory; J data_store_memory; l data_store_memory; pi data_store_memory; kp data_store_memory; ki data_store_memory; k1 data_store_memory; k2 data_store_memory; k3 data_store_memory; kd data_store_memory
function y = fcn(e,s,de,dA,dt,ddAr)
global J l pi kp ki kd k1 k2 k3;

y =-dt/l+J*ddAr+J/kd*(kp*de+ki*k1*tanh(e)+k2*s+k3*sign(s));

== matlab function Trajactory_uav/Subsystem/MATLAB Function ==
  settings: updateMethod=DISCRETE
  data: e input; y output; de input; inte input; kp data_store_memory; ki data_store_memory; kd data_store_memory; k1 data_store_memory
function y = fcn(e,de,inte)
global kp;
global ki;
global kd;
global k1;

y = kp*e+ki*k1*inte+kd*de;

== matlab function Trajactory_uav/Subsystem7/MATLAB Function ==
  settings: updateMethod=DISCRETE
  data: e input; y output; de input; inte input; kp1 data_store_memory; ki1 data_store_memory; kd1 data_store_memory; k11 data_store_memory
function y = fcn(e,de,inte)
global kp1;
global ki1;
global kd1;
global k11;

y = kp1*e+ki1*k11*inte+kd1*de;

== matlab function Trajactory_uav/Subsystem9/MATLAB Function ==
  settings: updateMethod=DISCRETE
  data: e input; s input; y output; de input; dA input; dt input; ddAr input; K0 data_store_memory; J1 data_store_memory; l data_store_memory; pi data_store_memory; k21 data_store_memory; k31 data_store_memory; kp1 data_store_memory; ki1 data_store_memory; kd1 data_store_memory; k11 data_store_memory
function y = fcn(e,s,de,dA,dt,ddAr)
global J1 l pi kp1 ki1 kd1 k11 k21 k31;

y =-dt/l+J1*ddAr+J1/kd1*(kp1*de+ki1*k11*tanh(e)+k21*s+k31*sign(s));

== matlab function Trajactory_uav/x-slider-surface/MATLAB Function ==
  settings: updateMethod=DISCRETE
  data: e input; y output; de input; inte input; xkp data_store_memory; xki data_store_memory; xkd data_store_memory; xk1 data_store_memory
function y = fcn(e,de,inte)
global xkp;
global xki;
global xkd;
global xk1;

y = xkp*e+xki*xk1*inte+xkd*de;
